simulink model "ElectricCircuitEquivalentModel"  (R2022b)
settings: Solver=ode4  StartTime=0.0  StopTime=25  FixedStep=0.0001  RelTol=1e-3
values from neighbouring files (symbols this model uses):
  Tsim = 1e-4    (= 0.0001)    [PAC_IV.m]
libraries: spsControlledCurrentSourceLib x4, spsSeriesRLCBranchLib x3, spsVoltageMeasurementLib x2, spsDCVoltageSourceLib x1, spsFuelCellStackLib x1, spsGroundLib x1, sps_lib x1
settings Model: Creator=ZinouAb  LastModifiedBy=ZinouAb

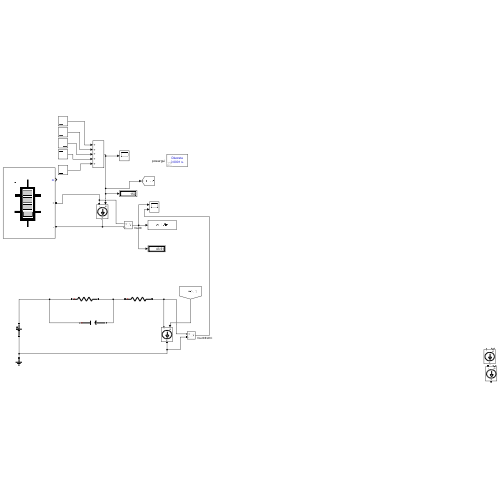
[thumbnail: Simulink's stored preview of the top-level diagram]
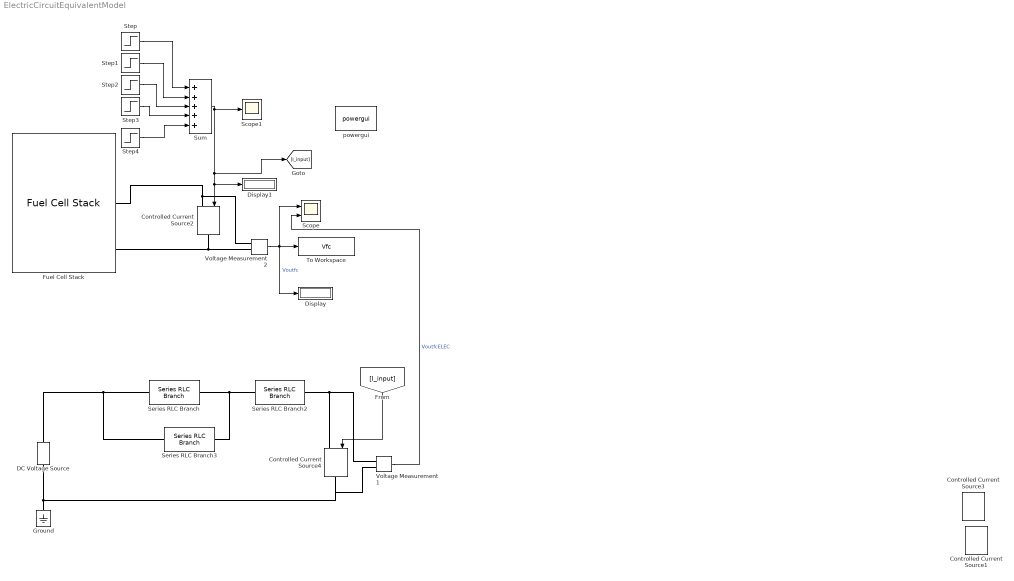
== system ElectricCircuitEquivalentModel ==
  Controlled Current Source{1..4} (4 alike) : spsControlledCurrentSourceLib/Controlled Current Source  Initialize=on  Source_Type=AC  Amplitude=0  Phase=0  Frequency=0  Measurements=None
  DC Voltage Source : spsDCVoltageSourceLib/DC Voltage Source  Amplitude=65  Measurements=None
  Display : Display
  Display1 : Display
  Fuel Cell Stack : spsFuelCellStackLib/Fuel Cell Stack  PresetModel=PEMFC - 6 kW - 45 Vdc  FcType=Proton Exchange Membrane (PEM)  Detailed=Detailed  Eoc=[65,63]  NomVI=[133.3,45]  EndVI=[225,37]  Nc=65  n=55  TOp=65  AirFr=300  SuppPress=[1.5,1]  Comp=[99.95,21,1]  SignX=off  SignY=off  FlowRateH2=off  FlowRateAir=off  SystemTemp=off  SystemPH2=off  SystemPAir=off  FCDyn=on  FC_tau=0.5  Peak_O2=80  V_Under=10
      settings: LibrarySourceBlock=electricdrivelib/Extra Sources/Fuel Cell Stack
  Ground : spsGroundLib/Ground  LConnTagsString=a
  Scope : Scope  NumInputPorts=2
  Scope1 : Scope
  Series RLC Branch : spsSeriesRLCBranchLib/Series RLC Branch  LConnTagsString=__new0  RConnTagsString=__new0  BranchType=R  Resistance=0.0914  Inductance=1e-3  SetiL0=off  InitialCurrent=0  Capacitance=1e-6  Setx0=off  InitialVoltage=0  Measurements=None
  Series RLC Branch2 : spsSeriesRLCBranchLib/Series RLC Branch  LConnTagsString=__new0  RConnTagsString=__new0  BranchType=R  Resistance=0.07833  Inductance=1e-3  SetiL0=off  InitialCurrent=0  Capacitance=1e-6  Setx0=off  InitialVoltage=0  Measurements=None
  Series RLC Branch3 : spsSeriesRLCBranchLib/Series RLC Branch  LConnTagsString=__new0  RConnTagsString=__new0  BranchType=C  Resistance=1  Inductance=1e-3  SetiL0=off  InitialCurrent=0  Capacitance=0.5/(0.0914)  Setx0=off  InitialVoltage=0  Measurements=None
  Step : Step  Before=70  After=100  SampleTime=0
  Step1 : Step  Time=7  After=30  SampleTime=0
  Step2 : Step  Time=10  After=-30  SampleTime=0
  Step3 : Step  Time=15  After=-40  SampleTime=0
  Step4 : Step  Time=20  After=+90  SampleTime=0
  Sum : Sum  Inputs=+++++
  To Workspace : ToWorkspace  VariableName=Vfc  SaveFormat=Timeseries  SampleTime=-1
  Voltage Measurement1 : spsVoltageMeasurementLib/Voltage Measurement  PhasorSimulation=off  OutputType=Complex  PSBequivalent=0
  Voltage Measurement2 : spsVoltageMeasurementLib/Voltage Measurement  PhasorSimulation=off  OutputType=Complex  PSBequivalent=0
  powergui : sps_lib/powergui  Priority=1  SimulationMode=Discrete  SampleTime=Tsim  frequency=60  Iterations=50  frequencyindice=0  Pbase=100e6  ErrMax=1e-4  UnitsV=kV  UnitsW=MW  buscounter=0  FunctionMessages=off  echomessages=off  EnableUseOfTLC=off  CurrentSourceSwitches=off  DisableSnubberDevices=on  DisableRonSwitches=on  DisableVfSwitches=on  DisplayEquations=off  AutomaticDiscreteSolvers=off  SolverType=Tustin  Interpol=off  ExternalGateDelay=off  methode=off  Ts=0  x0status=blocks  SPID=on  SwTol=0  HookPort=off  NonlinearTolerance=1e-4  nMaxIteration=100  ContinueOnMaxIteration=off  RestoreLinks=warning  ResistiveCurrentMeasurement=off  Frange=[0:2:500]  Ylog=off  Xlog=on  ShowGrid=off  save=off  variable=ZData  structure=0  ZoomFFT=off  StartTime=0.0  cycles=1  DisplayStyle=1  fundamental=60  FreqAxis=off  MaxFrequency=1000  frequencyindicesteady=1  RmsSteady=1  display=off
  wires:
  Sum/1 -> Scope1/1, Display1/1, Controlled Current Source2/1, [I_input]
  Voltage Measurement2/1 -> Display/1, Scope/1, To Workspace/1  "Voutfc"
  [I_input] -> Controlled Current Source4/1
  Voltage Measurement1/1 -> Scope/2  "VoutfcELEC"
  Step1/1 -> Sum/2
  Step2/1 -> Sum/3
  Step/1 -> Sum/1
  Step3/1 -> Sum/4
  Step4/1 -> Sum/5
  connections:
  Voltage Measurement2/LConn1 -- Controlled Current Source2/LConn1 -- Fuel Cell Stack/RConn1
  Voltage Measurement2/LConn2 -- Controlled Current Source2/RConn1 -- Fuel Cell Stack/RConn2
  DC Voltage Source/RConn1 -- Series RLC Branch3/LConn1 -- Series RLC Branch/LConn1
  Series RLC Branch3/RConn1 -- Series RLC Branch2/LConn1 -- Series RLC Branch/RConn1
  Ground/LConn1 -- Voltage Measurement1/LConn2 -- Controlled Current Source4/RConn1 -- DC Voltage Source/LConn1
  Controlled Current Source4/LConn1 -- Voltage Measurement1/LConn1 -- Series RLC Branch2/RConn1
